simulink model "PDdecouple - 副本"  (R2021b)
settings: Solver=FixedStepAuto  StartTime=0.0  StopTime=5  FixedStep=1e-3  MaxStep=1e-2  RelTol=1e-5  AbsTol=1e-6
values from neighbouring files (symbols this model uses):
  gravity = [0;0;-9.81]    [parameters.m]
  Inertia = [5.5*10^(-7) 0 0;0 5.5*10^(-7) 0;0 0 11*10^(-7)]    [parameters.m]
  kd = 10    [parameters.m]
  kp = 10    [parameters.m]
  kq = 1000    [parameters.m]
  kw = 50    [parameters.m]
  mass = 0.027    [parameters.m]
libraries: simulink x4, Contact_Forces_Lib x2, sharedutil x1, sharedtransform x1
settings Model: Creator=thinkpad  LastModifiedBy=thinkpad

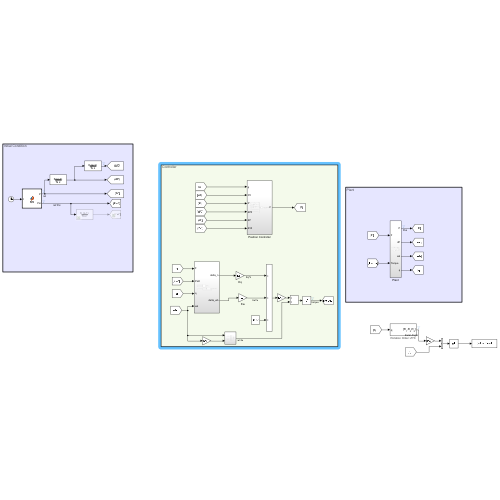
[thumbnail: Simulink's stored preview of the top-level diagram]
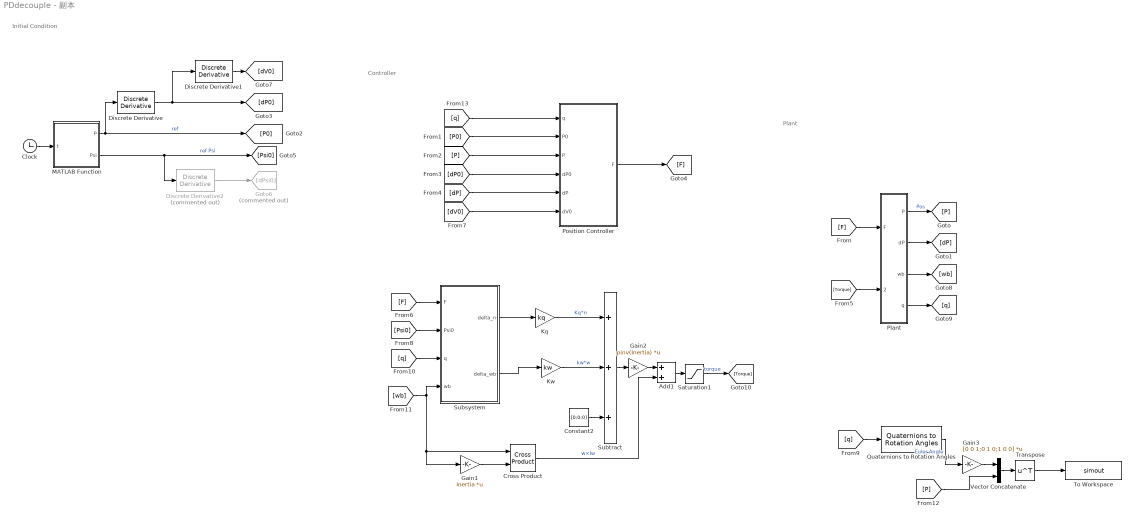
== system PDdecouple - 副本 ==
  note: Controller
  note: Initial Condition
  note: Plant
  Add1 : Sum
  Clock : Clock
  Constant2 : Constant  Value=[0;0;0]
  Cross Product : Contact_Forces_Lib/Math/Cross Product  SystemSampleTime=-1  VariantActivationTime=update diagram  Latency=0  AutoFrameSizeCalculation=off
      settings: SourceProductName=Simscape Multibody Contact Forces Library
  Discrete Derivative : simulink/Discrete/Discrete Derivative  gainval=1.0  ICPrevScaledInput=0.0  OutMin=[]  OutMax=[]  OutDataType=fixdt(1, 16)  OutScaling=2^-10  DoSatur=off
  Discrete Derivative1 : simulink/Discrete/Discrete Derivative  gainval=1.0  ICPrevScaledInput=0.0  OutMin=[]  OutMax=[]  OutDataType=fixdt(1, 16)  OutScaling=2^-10  DoSatur=off
  Discrete Derivative2 : simulink/Discrete/Discrete Derivative  Commented=on  gainval=1.0  ICPrevScaledInput=0.0  OutMin=[]  OutMax=[]  OutDataType=fixdt(1, 16)  OutScaling=2^-10  DoSatur=off
  Gain1 : Gain  Gain=Inertia  Multiplication=Matrix(K*u)
  Gain2 : Gain  Gain=pinv(Inertia)  Multiplication=Matrix(K*u)
  Gain3 : Gain  Gain=[0 0 1;0 1 0;1 0 0]  Multiplication=Matrix(K*u)
  Goto6 : Goto  Commented=on  GotoTag=dPsi0
  Kq : Gain  Gain=kq
  Kw : Gain  Gain=kw
  MATLAB Function : MATLAB Function  TreatAsAtomicUnit=on
  Plant : Subsystem
  Position Controller : Subsystem
  Quaternions to Rotation Angles : sharedtransform/Quaternions to Rotation Angles  rotationOrder=ZYX  aMode=aMode
      settings: SourceProductBaseCode=AE,PW,DR,MT,UV,VE
  Saturation1 : Saturate  UpperLimit=[0.1;0.1;0.1]  LowerLimit=[-0.1;-0.1;-0.1]
  Subsystem : Subsystem
  Subtract : Sum  Inputs=+++
  To Workspace : ToWorkspace  VariableName=simout  SampleTime=-1
      settings: Save2DSignal=2-D array (concatenate along first dimension)
  Transpose : Math  Operator=transpose  SaturateOnIntegerOverflow=on
  Vector Concatenate : Concatenate
  wires:
  Plant/2(dP) -> [dP]
  Plant/1(P) -> [P]  "Pos"
  [F] -> Plant/1(F)
  MATLAB Function/1(P) -> [P0], Discrete Derivative/1  "ref"
  Discrete Derivative1/1 -> [dV0]
  Clock/1 -> MATLAB Function/1(t)
  Discrete Derivative/1 -> [dP0], Discrete Derivative1/1
  MATLAB Function/2(Psi) -> Discrete Derivative2/1, [Psi0]  "ref Psi"
  Discrete Derivative2/1 -> Goto6/1
  Plant/3(wb) -> [wb]
  Plant/4(q) -> [q]
  [Torque] -> Plant/2(Torque)
  Gain1/1 -> Cross Product/2
  [F] -> Subsystem/1(F)
  [Psi0] -> Subsystem/2(Psi0)
  [q] -> Subsystem/3(q)
  [wb] -> Cross Product/1, Gain1/1, Subsystem/4(wb)
  Subsystem/1(delta_n) -> Kq/1
  Subsystem/2(delta_wb) -> Kw/1
  [q] -> Quaternions to Rotation Angles/1
  Quaternions to Rotation Angles/1 -> Gain3/1  "Euler Angle"
  Gain3/1 -> Vector Concatenate/1
  Vector Concatenate/1 -> Transpose/1
  [P] -> Vector Concatenate/2
  Transpose/1 -> To Workspace/1
  Saturation1/1 -> [Torque]  "torque"
  Cross Product/1 -> Add1/2  "w×Iw"
  Add1/1 -> Saturation1/1
  Subtract/1 -> Gain2/1
  Gain2/1 -> Add1/1
  Kw/1 -> Subtract/2  "kw*w"
  Constant2/1 -> Subtract/3
  Kq/1 -> Subtract/1  "Kq*n"
  [q] -> Position Controller/1(q)
  [P0] -> Position Controller/2(P0)
  [dP0] -> Position Controller/4(dP0)
  [dV0] -> Position Controller/6(dV0)
  Position Controller/1(F) -> [F]
  [P] -> Position Controller/3(P)
  [dP] -> Position Controller/5(dP)

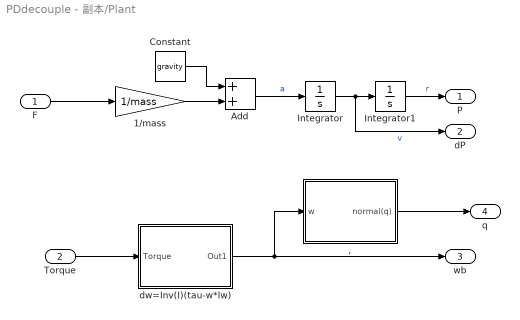
== system PDdecouple - 副本/Plant ==
  F : Inport
  Torque : Inport  Port=2  PortDimensions=3
  , : Subsystem
  1/mass : Gain  Gain=1/mass
  Add : Sum
  Constant : Constant  Value=gravity
  Integrator : Integrator  InitialCondition=[0;0;0]
  Integrator1 : Integrator  InitialCondition=[0;0;0]
  dw=Inv(I)(tau-w*Iw) : Subsystem
  P : Outport
  dP : Outport  Port=2
  wb : Outport  Port=3
  q : Outport  Port=4
  wires:
  Integrator1/1 -> P/1  "r"
  Constant/1 -> Add/1
  Integrator/1 -> Integrator1/1, dP/1  "v"
  1/mass/1 -> Add/2
  Add/1 -> Integrator/1  "a"
  dw=Inv(I)(tau-w*Iw)/1(Out1) -> wb/1, ,/1(w)
  Torque/1 -> dw=Inv(I)(tau-w*Iw)/1(Torque)
  F/1 -> 1/mass/1
  ,/1(normal(q)) -> q/1

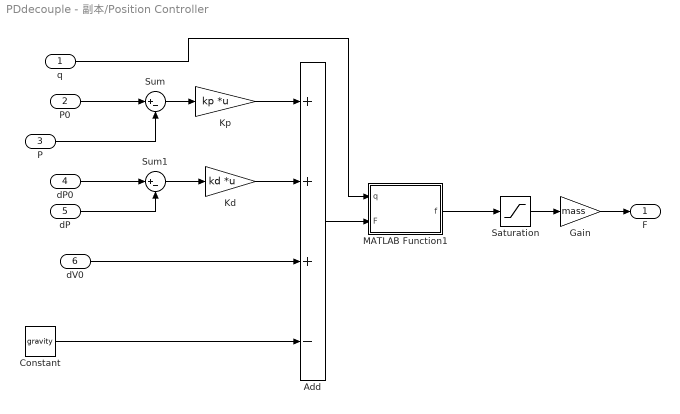
== system PDdecouple - 副本/Position Controller ==
  q : Inport
  P0 : Inport  Port=2
  P : Inport  Port=3
  dP0 : Inport  Port=4
  dP : Inport  Port=5
  dV0 : Inport  Port=6
  Add : Sum  Inputs=+++-
  Constant : Constant  Value=gravity
  Gain : Gain  Gain=mass
  Kd : Gain  Gain=kd  Multiplication=Matrix(K*u)
  Kp : Gain  Gain=kp  Multiplication=Matrix(K*u)
  MATLAB Function1 : MATLAB Function  TreatAsAtomicUnit=on
  Saturation : Saturate  UpperLimit=[30;30;30]  LowerLimit=[-30;-30;-9.81]
  Sum : Sum  Inputs=|+-
  Sum1 : Sum  Inputs=|+-
  F : Outport
  wires:
  P/1 -> Sum/2
  Kp/1 -> Add/1
  dP/1 -> Sum1/2
  Sum/1 -> Kp/1
  Sum1/1 -> Kd/1
  Kd/1 -> Add/2
  Saturation/1 -> Gain/1
  q/1 -> MATLAB Function1/1(q)
  dP0/1 -> Sum1/1
  dV0/1 -> Add/3
  Constant/1 -> Add/4
  P0/1 -> Sum/1
  Gain/1 -> F/1
  MATLAB Function1/1(f) -> Saturation/1
  Add/1 -> MATLAB Function1/2(F)

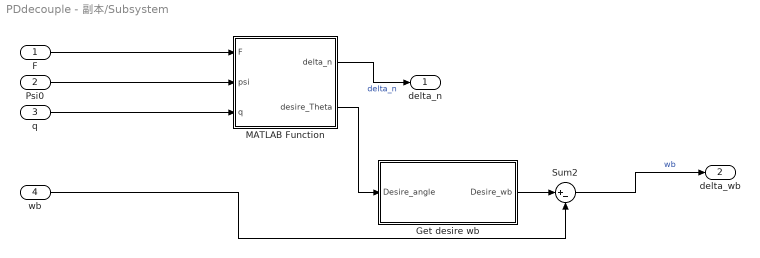
== system PDdecouple - 副本/Subsystem ==
  F : Inport
  Psi0 : Inport  Port=2
  q : Inport  Port=3
  wb : Inport  Port=4
  Get desire wb : Subsystem
  MATLAB Function : MATLAB Function  TreatAsAtomicUnit=on
  Sum2 : Sum  Inputs=|+-
  delta_n : Outport
  delta_wb : Outport  Port=2
  wires:
  wb/1 -> Sum2/2
  Get desire wb/1(Desire_wb) -> Sum2/1
  q/1 -> MATLAB Function/3(q)
  MATLAB Function/1(delta_n) -> delta_n/1  "delta_n"
  Psi0/1 -> MATLAB Function/2(psi)
  F/1 -> MATLAB Function/1(F)
  MATLAB Function/2(desire_Theta) -> Get desire wb/1(Desire_angle)
  Sum2/1 -> delta_wb/1  "wb"

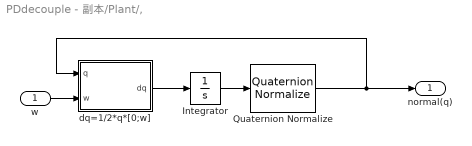
== system PDdecouple - 副本/Plant/, ==
  w : Inport
  Integrator : Integrator  InitialCondition=[1;0;0;0]
  Quaternion Normalize : sharedutil/Quaternion Normalize  aMode=aMode
      settings: SourceProductBaseCode=AE,PW,DR,MT,UV,VE
  dq=1/2*q*[0;w] : MATLAB Function  TreatAsAtomicUnit=on
  normal(q) : Outport
  wires:
  Quaternion Normalize/1 -> dq=1/2*q*[0;w]/1(q), normal(q)/1
  Integrator/1 -> Quaternion Normalize/1
  dq=1/2*q*[0;w]/1(dq) -> Integrator/1
  w/1 -> dq=1/2*q*[0;w]/2(w)

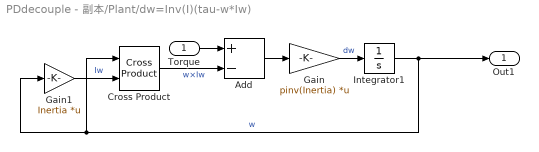
== system PDdecouple - 副本/Plant/dw=Inv(I)(tau-w*Iw) ==
  Torque : Inport  PortDimensions=3
  Add : Sum  Inputs=+-
  "Cross Product " : Contact_Forces_Lib/Math/Cross Product  SystemSampleTime=-1  VariantActivationTime=update diagram  Latency=0  AutoFrameSizeCalculation=off
      settings: SourceProductName=Simscape Multibody Contact Forces Library
  Gain : Gain  Gain=pinv(Inertia)  Multiplication=Matrix(K*u) (u vector)
  Gain1 : Gain  Gain=Inertia  Multiplication=Matrix(K*u)
  Integrator1 : Integrator  InitialCondition=[0;0;0]
  Out1 : Outport
  wires:
  Gain/1 -> Integrator1/1  "dw"
  "Cross Product "/1 -> Add/2  "w×Iw"
  Integrator1/1 -> Out1/1, Gain1/1, "Cross Product "/1  "w"
  Add/1 -> Gain/1
  Gain1/1 -> "Cross Product "/2  "Iw"
  Torque/1 -> Add/1

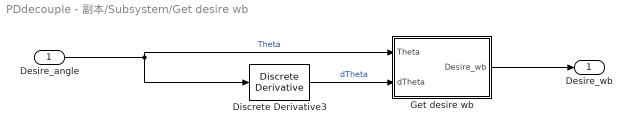
== system PDdecouple - 副本/Subsystem/Get desire wb ==
  Desire_angle : Inport
  Discrete Derivative3 : simulink/Discrete/Discrete Derivative  gainval=1.0  ICPrevScaledInput=0.0  OutMin=[]  OutMax=[]  OutDataType=fixdt(1, 16)  OutScaling=2^-10  DoSatur=off
  Get desire wb : MATLAB Function  TreatAsAtomicUnit=on
  Desire_wb : Outport
  wires:
  Discrete Derivative3/1 -> Get desire wb/2(dTheta)  "dTheta"
  Desire_angle/1 -> Get desire wb/1(Theta), Discrete Derivative3/1  "Theta"
  Get desire wb/1(Desire_wb) -> Desire_wb/1

== matlab function PDdecouple - 副本/Subsystem/Get desire wb/Get desire wb ==
  data: Theta input size=3; Desire_wb output size=3; dTheta input size=3
function Desire_wb = T_dTheta(Theta, dTheta)
row=Theta(1);
pitch=Theta(2);
yaw=Theta(3);
T=[cos(pitch)*cos(yaw) -sin(yaw) 0;cos(pitch)*sin(yaw) cos(yaw) 0;-sin(pitch) 0 1];
Desire_wb=T*dTheta;
end

== matlab function PDdecouple - 副本/MATLAB Function ==
  data: t input; P output; Psi output
function [P,Psi] = fcn(t)
x=cos(t)-1+1;
y=sin(t)+1;
z=1-exp(-t)+1;
% P=[x;y;z];
P=[0;0;0];
Psi=1-exp(-t);
% Psi=0;
end

== matlab function PDdecouple - 副本/Plant/,/dq=1//2*q*[0;w] ==
  data: q input; dq output; w input
function dq = fcn(q,w)
dq=1/2*quatmultiply(q.',[0 w.']);
end

== matlab function PDdecouple - 副本/Subsystem/MATLAB Function ==
  data: delta_n output size=3; F input size=3; psi input size=1; q input size=4; desire_Theta output
function [delta_n, desire_Theta] = fcn(F, psi, q)
coder.extrinsic('dcm2angle');
coder.extrinsic('dcm2quat');
f= norm(F);
if f==0
    %R=[cos(psi) -sin(psi) 0; sin(psi) cos(psi) 0;0 0 1];
    desire_Theta=[0;0;psi];
    q0=[cos(psi/2) 0 0 sin(psi/2)];

else
    u3=F./f;
    u1=[cos(psi);sin(psi);0];
    u2=cross(u3,u1);
    u2=u2./norm(u2);
    u1=cross(u2,u3);
    Rt=[u1 u2 u3];
    q0=dcm2quat(Rt.');
    desire_Theta=zeros(3,1);
     [desire_Theta(3),desire_Theta(2),desire_Theta(1)]=dcm2angle(Rt.');
end
    delta_q=QuatDivide(q0,q.');
    delta_n=delta_q(2:4);
   
end

== matlab function PDdecouple - 副本/Position Controller/MATLAB Function1 ==
  data: q input; f output; F input
function f = fcn(q,F)

Zaxis=QuatRotation(q,[0 0 0 1]);
f=F.*Zaxis(2:4);
end
